simulink library "cjt_library_models"  (Simulink 8.9)
settings: Solver=ode45  StartTime=0.0  StopTime=10.0  RelTol=1e-3  EnableMultiTasking=on
undefined symbols (not defined in the file or in its folder): A, B, C, D, jointObj
libraries: simulink x7, cstblocks x4, cjt_library_models x2
settings Model: SuppressorTable=22 serialization::archive 11 0 6 0 0 0 11 0  Creator=wesley  LastModifiedBy=wesley

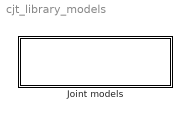
== system cjt_library_models ==
  Joint models : Subsystem

== system cjt_library_models/Joint models ==
  note: Electrical Models
  note: Mechanical Models
  JointElectricalSubsystem : Subsystem  mask{jointObj=jointObj, input_delay=0, quantize=off, quantize_bits=32, input_noise_enabled=off, var_u=0.12}
      mask prompts: jointObj "Joint Object"; input_delay "Input Delay (num samples)"; quantize "Quantize input"; quantize_bits "Quantization bits"; input_noise_enabled "Enable input noise"; var_u "Input Noise Variance"
      mask init:
      | % Get linear dynamics matrices
      | [A, B, C, D] = jointObj.getElectricalDynamicsMatrices();
      | 
      | % Get other properties
      | Ts      = jointObj.Ts;
      | Ts_elec = jointObj.Ts_elec;
      | 
      | % If noise is disabled, overwrite the given variances
      | if (input_noise_enabled == 0)
      |     var_u = 0;
      | end
      mask Callback quantize: toggleMaskFields(gcbh, 'quantize', 'quantize_bits');
      mask Callback input_noise_enabled: toggleMaskFields(gcbh, 'input_noise_enabled', 'var_u');
  JointElectricalSubsystem with d-q axes : Subsystem  mask{jointObj=jointObj, input_delay=0, quantize=off, quantize_bits=32, input_noise_enabled=off, var_u=0.0013}
      mask prompts: jointObj "Joint Object"; input_delay "Input Delay (num samples)"; quantize "Quantize input"; quantize_bits "Quantization bits"; input_noise_enabled "Enable input noise"; var_u "Input Noise Variance"
      mask init:
      | % Get other properties
      | Ts      = jointObj.Ts;
      | Ts_elec = jointObj.Ts_elec;
      | 
      | % If noise is disabled, overwrite the given variances
      | if (input_noise_enabled == 0)
      |     var_u = 0;
      | end
      mask Callback quantize: toggleMaskFields(gcbh, 'quantize', 'quantize_bits');
      mask Callback input_noise_enabled: toggleMaskFields(gcbh, 'input_noise_enabled', 'var_u');
  JointMechanicalSubsystem : Subsystem  mask{jointObj=jointObj, fc_vel=200, fc_torque=200, input_delay=1, output_delay=1, quantize=on, quantize_bits=19, input_noise_enabled=on, output_noise_enabled=on, var_u=0.12^2, var_y=1.8e-10}
      mask prompts: jointObj "Joint Object"; fc_vel "Velocity filter cut-off frequency [Hz]"; fc_torque "Torque filter cut-off frequency [Hz]"; input_delay "Input delay (num samples)"; output_delay "Output delay (num samples)"; quantize "Quantize measurements"; quantize_bits "Quantization bits"; input_noise_enabled "Enable input noise"; output_noise_enabled "Enable measurement noise"; var_u "Input noise variance"; var_y "Measurement noise variance"
      mask init:
      | % Get linear dynamics matrices
      | [A, B, C, D, I, R, K] = jointObj.getDynamicsMatrices();
      | 
      | % Build B matrix for nonlinear components
      | B_nonlinear = [zeros([size(B,1)-size(I,1),1]); 1./diag(I)];
      | 
      | % Get other properties
      | Ts      = jointObj.Ts;
      | Ts_elec = jointObj.Ts_elec;
      | k_b     = jointObj.k_b;
      | k_t     = jointObj.k_t;
      | n       = jointObj.n;
      | 
      | % Handle MATLAB function block
      | handleMatlabFunctionBlock(gcb, jointObj);
      | 
      | % If noise is disabled, overwrite the given variances
      | if (input_noise_enabled == 0)
      |     var_u = 0;
      | end
      | if (output_noise_enabled == 0)
      | 	var_y = 0;
      | end
      settings: ModelCloseFcn=sfsave  DestroyFcn=sfsave
      mask Callback quantize: toggleMaskFields(gcbh, 'quantize', 'quantize_bits');
      mask Callback input_noise_enabled: toggleMaskFields(gcbh, 'input_noise_enabled', 'var_u');
      mask Callback output_noise_enabled: toggleMaskFields(gcbh, 'output_noise_enabled', 'var_y');

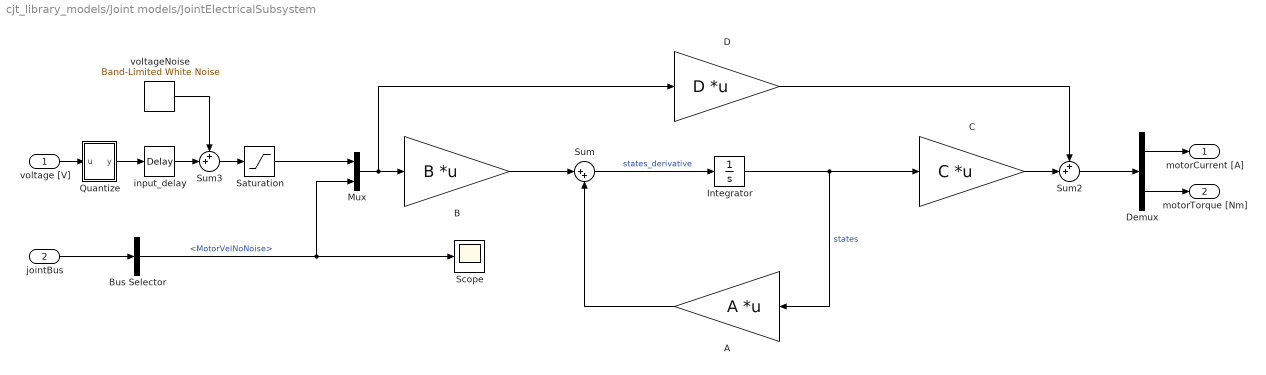
== system cjt_library_models/Joint models/JointElectricalSubsystem ==
  voltage [V] : Inport
  jointBus : Inport  Port=2
  A : Gain  Gain=A  Multiplication=Matrix(K*u)
  B : Gain  Gain=B  Multiplication=Matrix(K*u)
  Bus Selector : BusSelector  OutputSignals=MotorVelNoNoise
  C : Gain  Gain=C  Multiplication=Matrix(K*u)
  D : Gain  Gain=D  Multiplication=Matrix(K*u)
  Demux : Demux  Outputs=2
  Integrator : Integrator
  Mux : Mux  Inputs=2
  Quantize : Subsystem
  Saturation : Saturate  UpperLimit=jointObj.v_0  LowerLimit=-jointObj.v_0
  Scope : Scope
  Sum : Sum  Inputs=|++
  Sum2 : Sum  Inputs=++|
  Sum3 : Sum  Inputs=++|
  input_delay : TransportDelay  DelayTime=input_delay * Ts_elec  TransDelayFeedthrough=on
  voltageNoise : simulink/Sources/Band-Limited White Noise  Cov=var_u * Ts_elec  Ts=Ts_elec  seed=[2435345645]
  motorCurrent [A] : Outport
  motorTorque [Nm] : Outport  Port=2
  wires:
  input_delay/1 -> Sum3/2
  Quantize/1(y) -> input_delay/1
  Bus Selector/1 -> Mux/2, Scope/1  "<MotorVelNoNoise>"
  Sum3/1 -> Saturation/1
  voltageNoise/1 -> Sum3/1
  Sum/1 -> Integrator/1  "states_derivative"
  Integrator/1 -> C/1, A/1  "states"
  A/1 -> Sum/2
  Mux/1 -> D/1, B/1
  D/1 -> Sum2/1
  C/1 -> Sum2/2
  B/1 -> Sum/1
  Sum2/1 -> Demux/1
  jointBus/1 -> Bus Selector/1
  voltage [V]/1 -> Quantize/1(u)
  Saturation/1 -> Mux/1
  Demux/1 -> motorCurrent [A]/1
  Demux/2 -> motorTorque [Nm]/1

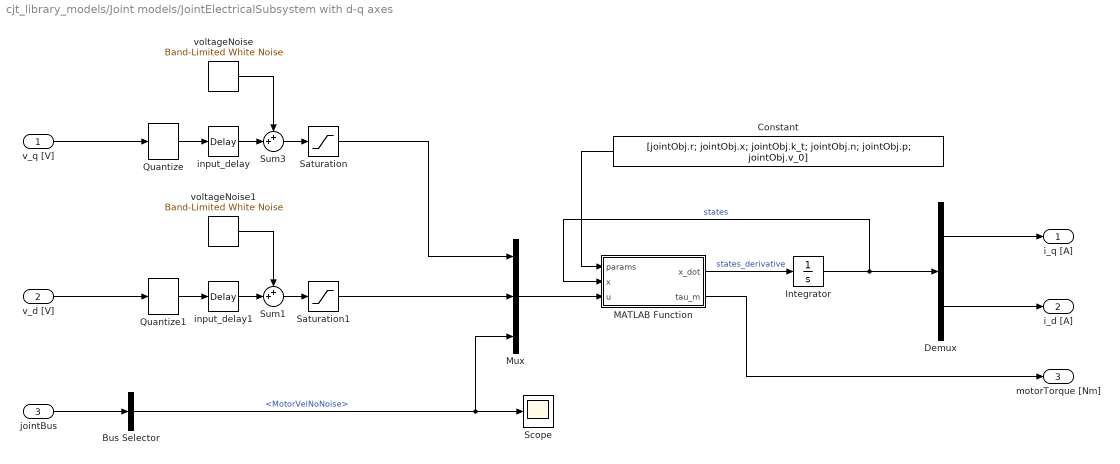
== system cjt_library_models/Joint models/JointElectricalSubsystem with d-q axes ==
  v_q [V] : Inport
  v_d [V] : Inport  Port=2
  jointBus : Inport  Port=3
  Bus Selector : BusSelector  OutputSignals=MotorVelNoNoise
  Constant : Constant  Value=[jointObj.r; jointObj.x; jointObj.k_t; jointObj.n; jointObj.p; jointObj.v_0]
  Demux : Demux  Outputs=2
  Integrator : Integrator  InitialCondition=[0;0]
  MATLAB Function : MATLAB Function  TreatAsAtomicUnit=on
  Mux : Mux  Inputs=3
  Quantize : cjt_library_models/Joint models/JointElectricalSubsystem/Quantize
  Quantize1 : cjt_library_models/Joint models/JointElectricalSubsystem/Quantize
  Saturation : Saturate  UpperLimit=jointObj.v_0  LowerLimit=-jointObj.v_0
  Saturation1 : Saturate  UpperLimit=jointObj.v_0  LowerLimit=-jointObj.v_0
  Scope : Scope
  Sum1 : Sum  Inputs=++|
  Sum3 : Sum  Inputs=++|
  input_delay : TransportDelay  DelayTime=input_delay * Ts_elec  TransDelayFeedthrough=on
  input_delay1 : TransportDelay  DelayTime=input_delay * Ts_elec  TransDelayFeedthrough=on
  voltageNoise : simulink/Sources/Band-Limited White Noise  Cov=var_u * Ts_elec  Ts=Ts_elec  seed=[2435345645]
  voltageNoise1 : simulink/Sources/Band-Limited White Noise  Cov=var_u * Ts_elec  Ts=Ts_elec  seed=[2435345645]
  i_q [A] : Outport
  i_d [A] : Outport  Port=2
  motorTorque [Nm] : Outport  Port=3
  wires:
  input_delay/1 -> Sum3/2
  Quantize/1 -> input_delay/1
  Bus Selector/1 -> Mux/3, Scope/1  "<MotorVelNoNoise>"
  Sum3/1 -> Saturation/1
  voltageNoise/1 -> Sum3/1
  MATLAB Function/1(x_dot) -> Integrator/1  "states_derivative"
  Integrator/1 -> MATLAB Function/2(x), Demux/1  "states"
  Mux/1 -> MATLAB Function/3(u)
  jointBus/1 -> Bus Selector/1
  v_q [V]/1 -> Quantize/1
  Saturation/1 -> Mux/1
  Demux/1 -> i_q [A]/1
  Demux/2 -> i_d [A]/1
  voltageNoise1/1 -> Sum1/1
  Sum1/1 -> Saturation1/1
  Quantize1/1 -> input_delay1/1
  input_delay1/1 -> Sum1/2
  v_d [V]/1 -> Quantize1/1
  Saturation1/1 -> Mux/2
  Constant/1 -> MATLAB Function/1(params)
  MATLAB Function/2(tau_m) -> motorTorque [Nm]/1

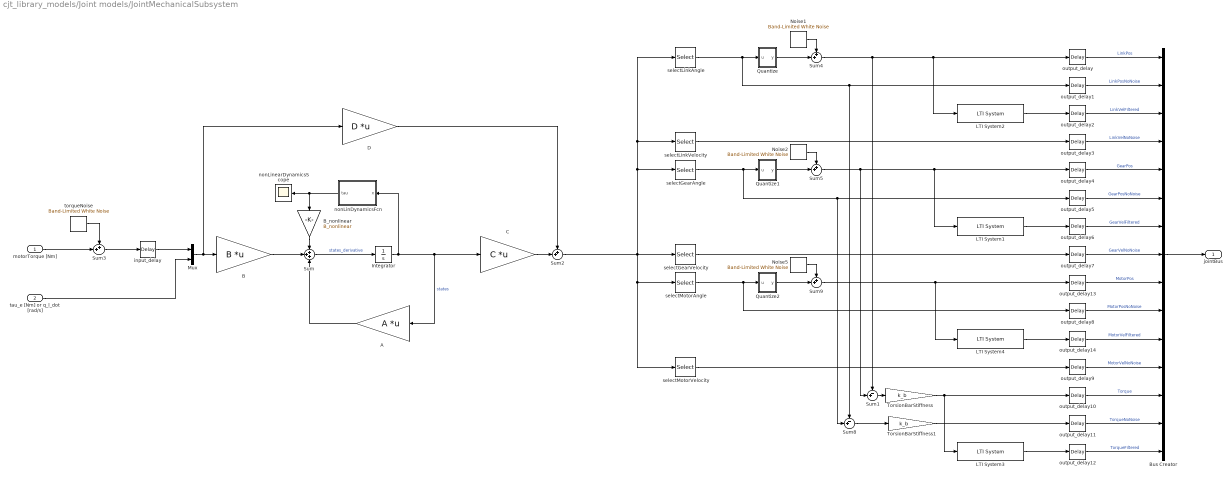
== system cjt_library_models/Joint models/JointMechanicalSubsystem ==
  motorTorque [Nm] : Inport
  tau_e [Nm] or q_l_dot [rad/s] : Inport  Port=2
  A : Gain  Gain=A  Multiplication=Matrix(K*u)
  B : Gain  Gain=B  Multiplication=Matrix(K*u)
  B_nonlinear : Gain  Gain=B_nonlinear
  Bus Creator : BusCreator  Inputs=15
  C : Gain  Gain=C  Multiplication=Matrix(K*u)
  D : Gain  Gain=D  Multiplication=Matrix(K*u)
  Integrator : Integrator
  LTI System1 : cstblocks/LTI System  sys=c2d(tf([2*pi*fc_vel 0], [1 2*pi*fc_vel]), Ts, 'tustin')  IC=[]
  LTI System2 : cstblocks/LTI System  sys=c2d(tf([2*pi*fc_vel 0], [1 2*pi*fc_vel]), Ts, 'tustin')  IC=[]
  LTI System3 : cstblocks/LTI System  sys=c2d(tf([2*pi*fc_torque], [1 2*pi*fc_torque]), Ts, 'tustin')  IC=[]
  LTI System4 : cstblocks/LTI System  sys=c2d(tf([2*pi*fc_vel 0], [1 2*pi*fc_vel]), Ts, 'tustin')  IC=[]
  Mux : Mux  Inputs=2
  Noise1 : simulink/Sources/Band-Limited White Noise  Cov=var_y * Ts  Ts=Ts  seed=[3846513]
  Noise2 : simulink/Sources/Band-Limited White Noise  Cov=var_y * Ts  Ts=Ts  seed=[11563454]
  Noise5 : simulink/Sources/Band-Limited White Noise  Cov=var_y * Ts  Ts=Ts  seed=[24326]
  Quantize : Subsystem
  Quantize1 : Subsystem
  Quantize2 : Subsystem
  Sum : Sum  Inputs=+++
  Sum1 : Sum  Inputs=-+|
  Sum{2..5,9} (5 alike) : Sum  Inputs=++|
  Sum8 : Sum  Inputs=-+|
  TorsionBarStiffness : Gain  Gain=k_b
  TorsionBarStiffness1 : Gain  Gain=k_b
  input_delay : TransportDelay  DelayTime=input_delay * jointObj.Ts  TransDelayFeedthrough=on
  nonLinDynamicsFcn : MATLAB Function  TreatAsAtomicUnit=on
  nonLinearDynamicsScope : Scope
  output_delay{,1..14} (15 alike) : TransportDelay  DelayTime=output_delay * jointObj.Ts
  selectGearAngle : Selector  NumberOfDimensions=2  InputPortWidth=3  IndexOptions=Index vector (dialog),Select all  Indices=2,1  OutputSizes=1,1
  selectGearVelocity : Selector  NumberOfDimensions=2  InputPortWidth=3  IndexOptions=Index vector (dialog),Select all  Indices=5,1  OutputSizes=1,1
  selectLinkAngle : Selector  NumberOfDimensions=2  InputPortWidth=3  IndexOptions=Index vector (dialog),Select all  Indices=3,1  OutputSizes=1,1
  selectLinkVelocity : Selector  NumberOfDimensions=2  InputPortWidth=3  IndexOptions=Index vector (dialog),Select all  Indices=6,1  OutputSizes=1,1
  selectMotorAngle : Selector  NumberOfDimensions=2  InputPortWidth=3  IndexOptions=Index vector (dialog),Select all  Indices=1,1  OutputSizes=1,1
  selectMotorVelocity : Selector  NumberOfDimensions=2  InputPortWidth=3  IndexOptions=Index vector (dialog),Select all  Indices=4,1  OutputSizes=1,1
  torqueNoise : simulink/Sources/Band-Limited White Noise  Cov=var_u * Ts  Ts=Ts  seed=[2435345645]
  jointBus : Outport
  wires:
  B_nonlinear/1 -> Sum/1
  nonLinDynamicsFcn/1(tau) -> nonLinearDynamicsScope/1, B_nonlinear/1
  Bus Creator/1 -> jointBus/1
  input_delay/1 -> Mux/1
  Sum3/1 -> input_delay/1
  Sum8/1 -> TorsionBarStiffness1/1
  Sum5/1 -> LTI System1/1, output_delay4/1, Sum1/2
  Sum4/1 -> LTI System2/1, output_delay/1, Sum1/1
  torqueNoise/1 -> Sum3/1
  Noise2/1 -> Sum5/1
  Noise1/1 -> Sum4/1
  selectMotorVelocity/1 -> output_delay9/1
  LTI System1/1 -> output_delay6/1
  selectGearVelocity/1 -> output_delay7/1
  Sum/1 -> Integrator/1  "states_derivative"
  selectLinkVelocity/1 -> output_delay3/1
  LTI System2/1 -> output_delay2/1
  motorTorque [Nm]/1 -> Sum3/2
  Sum1/1 -> TorsionBarStiffness/1
  Integrator/1 -> nonLinDynamicsFcn/1(x), C/1, A/1  "states"
  Sum2/1 -> selectGearVelocity/1, selectGearAngle/1, selectLinkVelocity/1, selectLinkAngle/1, selectMotorVelocity/1, selectMotorAngle/1
  B/1 -> Sum/2
  A/1 -> Sum/3
  output_delay/1 -> Bus Creator/1  "LinkPos"
  output_delay1/1 -> Bus Creator/2  "LinkPosNoNoise"
  output_delay2/1 -> Bus Creator/3  "LinkVelFiltered"
  output_delay3/1 -> Bus Creator/4  "LinkVelNoNoise"
  output_delay4/1 -> Bus Creator/5  "GearPos"
  output_delay5/1 -> Bus Creator/6  "GearPosNoNoise"
  output_delay6/1 -> Bus Creator/7  "GearVelFiltered"
  output_delay7/1 -> Bus Creator/8  "GearVelNoNoise"
  output_delay8/1 -> Bus Creator/10  "MotorPosNoNoise"
  output_delay9/1 -> Bus Creator/12  "MotorVelNoNoise"
  output_delay10/1 -> Bus Creator/13  "Torque"
  output_delay11/1 -> Bus Creator/14  "TorqueNoNoise"
  output_delay12/1 -> Bus Creator/15  "TorqueFiltered"
  Noise5/1 -> Sum9/1
  LTI System4/1 -> output_delay14/1
  output_delay13/1 -> Bus Creator/9  "MotorPos"
  output_delay14/1 -> Bus Creator/11  "MotorVelFiltered"
  Sum9/1 -> LTI System4/1, output_delay13/1
  Mux/1 -> D/1, B/1
  tau_e [Nm] or q_l_dot [rad/s]/1 -> Mux/2
  LTI System3/1 -> output_delay12/1
  TorsionBarStiffness1/1 -> output_delay11/1
  TorsionBarStiffness/1 -> output_delay10/1, LTI System3/1
  selectMotorAngle/1 -> output_delay8/1, Quantize2/1(u)
  selectGearAngle/1 -> output_delay5/1, Sum8/2, Quantize1/1(u)
  selectLinkAngle/1 -> Quantize/1(u), output_delay1/1, Sum8/1
  Quantize/1(y) -> Sum4/2
  Quantize1/1(y) -> Sum5/2
  Quantize2/1(y) -> Sum9/2
  D/1 -> Sum2/1
  C/1 -> Sum2/2

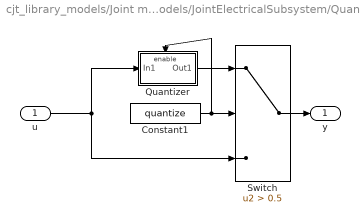
== system cjt_library_models/Joint models/JointElectricalSubsystem/Quantize ==
  u : Inport
  Constant1 : Constant  Value=quantize
  Quantizer : Subsystem
  Switch : Switch  Criteria=u2 > Threshold  Threshold=0.5
  y : Outport
  wires:
  u/1 -> Quantizer/1(In1), Switch/3
  Constant1/1 -> Quantizer/Enable, Switch/2
  Switch/1 -> y/1
  Quantizer/1(Out1) -> Switch/1

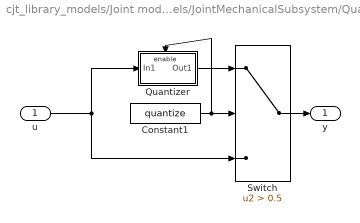
== system cjt_library_models/Joint models/JointMechanicalSubsystem/Quantize ==
  u : Inport
  Constant1 : Constant  Value=quantize
  Quantizer : Subsystem
  Switch : Switch  Criteria=u2 > Threshold  Threshold=0.5
  y : Outport
  wires:
  Quantizer/1(Out1) -> Switch/1
  Switch/1 -> y/1
  Constant1/1 -> Switch/2, Quantizer/Enable
  u/1 -> Switch/3, Quantizer/1(In1)

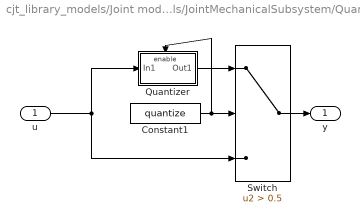
== system cjt_library_models/Joint models/JointMechanicalSubsystem/Quantize1 ==
  u : Inport
  Constant1 : Constant  Value=quantize
  Quantizer : Subsystem
  Switch : Switch  Criteria=u2 > Threshold  Threshold=0.5
  y : Outport
  wires:
  Quantizer/1(Out1) -> Switch/1
  Switch/1 -> y/1
  Constant1/1 -> Switch/2, Quantizer/Enable
  u/1 -> Switch/3, Quantizer/1(In1)

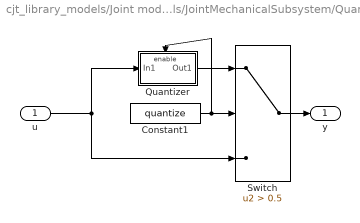
== system cjt_library_models/Joint models/JointMechanicalSubsystem/Quantize2 ==
  u : Inport
  Constant1 : Constant  Value=quantize
  Quantizer : Subsystem
  Switch : Switch  Criteria=u2 > Threshold  Threshold=0.5
  y : Outport
  wires:
  Quantizer/1(Out1) -> Switch/1
  Switch/1 -> y/1
  Constant1/1 -> Switch/2, Quantizer/Enable
  u/1 -> Switch/3, Quantizer/1(In1)

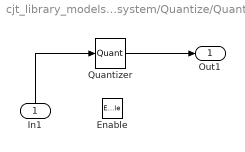
== system cjt_library_models/Joint models/JointElectricalSubsystem/Quantize/Quantizer ==
  In1 : Inport
  Enable : EnablePort
  Quantizer : Quantizer  QuantizationInterval=1/(2^quantize_bits)
  Out1 : Outport
  wires:
  In1/1 -> Quantizer/1
  Quantizer/1 -> Out1/1

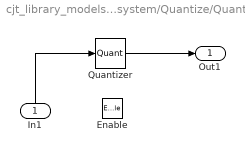
== system cjt_library_models/Joint models/JointMechanicalSubsystem/Quantize/Quantizer ==
  In1 : Inport
  Enable : EnablePort
  Quantizer : Quantizer  QuantizationInterval=1/(2^quantize_bits)
  Out1 : Outport
  wires:
  Quantizer/1 -> Out1/1
  In1/1 -> Quantizer/1

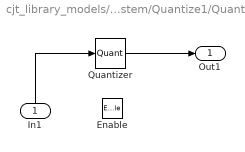
== system cjt_library_models/Joint models/JointMechanicalSubsystem/Quantize1/Quantizer ==
  In1 : Inport
  Enable : EnablePort
  Quantizer : Quantizer  QuantizationInterval=1/(2^quantize_bits)
  Out1 : Outport
  wires:
  Quantizer/1 -> Out1/1
  In1/1 -> Quantizer/1

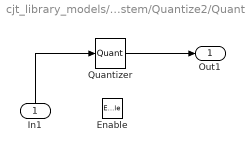
== system cjt_library_models/Joint models/JointMechanicalSubsystem/Quantize2/Quantizer ==
  In1 : Inport
  Enable : EnablePort
  Quantizer : Quantizer  QuantizationInterval=1/(2^quantize_bits)
  Out1 : Outport
  wires:
  Quantizer/1 -> Out1/1
  In1/1 -> Quantizer/1

== matlab function Joint models/JointElectricalSubsystem with d-q axes/MATLAB Function ==
  data: params input double; x input double; u input double; x_dot output double; tau_m output double
function [x_dot, tau_m] = fcn(params, x, u)
    [x_dot, tau_m] = electric_dyn_iq_id(params, x, u);

== matlab function Joint models/JointMechanicalSubsystem/nonLinDynamicsFcn ==
  data: x input double; tau output double
function tau = nonLinDynamics(x)
%#codegen

params.a_CU = 0.003900;
params.c_CU = 380.000000;
params.c_FE = 460.000000;
params.diam = 100.000000;
params.len = 150.000000;
params.m = 2.000000;
params.I_m = 0.216397;
params.I_g = 0.078848;
params.I_l = 1.000000;
params.k_g = 25000.000000;
params.k_b = 5714.000000;
params.d_m = 0.327578;
params.d_g = 2.235072;
params.d_l = 0.000010;
params.d_m_n = 0.327578;
params.d_g_n = 2.235072;
params.d_l_n = 0.000010;
params.d_mg = 300.000000;
params.d_gl = 5.000000;
params.d_cm = 2.640000;
params.d_cg = 2.320000;
params.d_cl = 0.020000;
params.d_cm_n = 2.640000;
params.d_cg_n = 2.320000;
params.d_cl_n = 0.020000;
params.d_s = 0.000000;
params.v_s = 0.000000;
params.rip_types = [];
params.rip_a1 = [];
params.rip_a2 = [];
params.rip_f = [];
params.n = 80.000000;
params.k_t = 0.078000;
params.r = 0.318000;
params.x = 0.000200;
params.p = 6.000000;
params.v_0 = 48.000000;
params.i_p = 0.000000;
params.dq_p = 0.000000;
params.r_th1 = 0.290000;
params.r_th2 = 3.450000;
params.T_thw = 3.960000;
params.T_thm = 1240.000000;
params.Tmp_WMax = 120.000000;
params.Tmp_ANom = 25.000000;
params.name = 'CE_Med_ds_rigid_gearbox_coulomb_torque_ripple';
params.paramName = 'CE_Med_ds';
params.modelName = 'rigid_gearbox';
%params.nonlinearModelName = {'coulomb', 'torque_ripple'}; % Cell arrays are not supported for code generation.
params.Ts = 0.001000;
params.Ts_elec = 0.000050;
tau =coulomb(params,x) +torque_ripple(params,x);
	end
